simulink library "bynary_asteroid"  (R2015a)
settings: Solver=ode45  StartTime=0.0  StopTime=10.0  RelTol=1e-3
undefined symbols (not defined in the file or in its folder): Target
libraries: vrlib x3, lib_gravity x2, RotationalDynamics x2, TranslationalDynamics3DoF x1
settings Model: Creator=bbrito  LastModifiedBy=bbrito

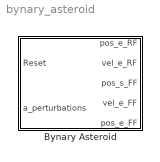
== system bynary_asteroid ==
  Bynary Asteroid : Subsystem  TreatAsAtomicUnit=on  mask{sphere=0, rt=0, ellip=0, sc=0, g=0, w0=0}
      mask prompts: sphere "Sphere parameters"; rt "Distance between bodies"; ellip "Ellipsoid parameters"; sc "Spacecraft initial conditions"; g "Gravitational constant"; w0 "Rotational speed"

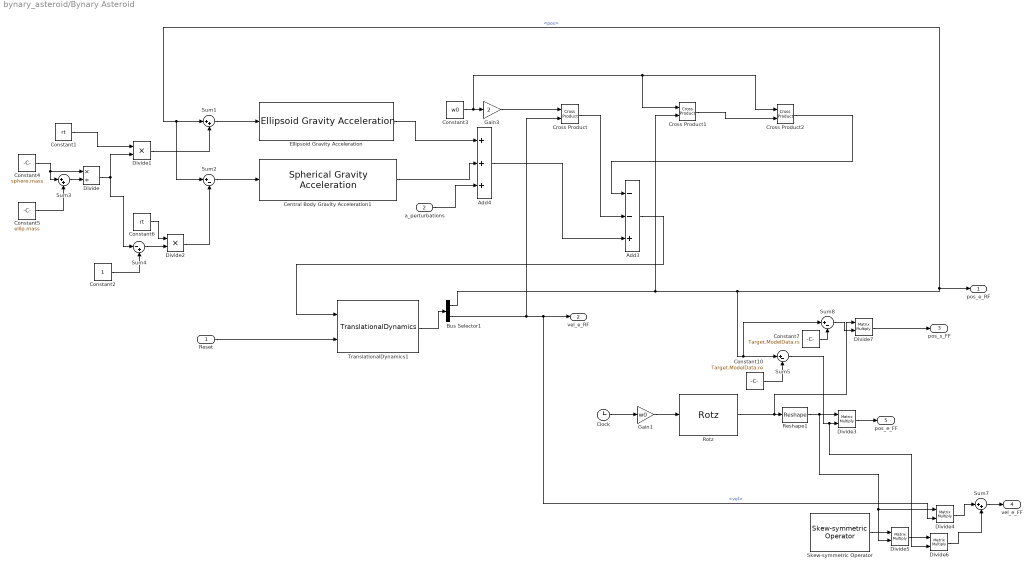
== system bynary_asteroid/Bynary Asteroid ==
  Reset : Inport
  a_perturbations : Inport  Port=2
  Add3 : Sum  Inputs=--+
  Add4 : Sum  Inputs=+++
  Bus Selector1 : BusSelector  OutputSignals=pos,vel
  Central Body Gravity Acceleration1 : lib_gravity/Spherical Gravity Acceleration  u=sphere.mass*g
  Clock : Clock
  Constant1 : Constant  Value=rt
  Constant10 : Constant  Value=Target.ModelData.re
  Constant2 : Constant
  Constant3 : Constant  Value=w0
  Constant4 : Constant  Value=sphere.mass
  Constant5 : Constant  Value=ellip.mass
  Constant6 : Constant  Value=rt
  Constant7 : Constant  Value=Target.ModelData.rs
  Cross Product : vrlib/Utilities/Cross Product
  Cross Product1 : vrlib/Utilities/Cross Product
  Cross Product2 : vrlib/Utilities/Cross Product
  Divide : Product  Inputs=*/
  Divide1 : Product  Inputs=**
  Divide2 : Product  Inputs=**
  Divide{3..7} (5 alike) : Product  Inputs=**  Multiplication=Matrix(*)
  Ellipsoid Gravity Acceleration : lib_gravity/Ellipsoid Gravity Acceleration  dim=ellip.dim  r0=ellip.r0  u=ellip.mass*g
  Gain1 : Gain  Gain=w0
  Gain3 : Gain  Gain=2
  Reshape1 : Reshape  OutputDimensionality=Customize  OutputDimensions=[3,3]
  Rotz : RotationalDynamics/Rotz
  Skew-symmetric Operator : RotationalDynamics/Skew-symmetric Operator  omega=Target.ModelData.Secondary.Rotation.w0
  Sum1 : Sum  Inputs=|++
  Sum2 : Sum  Inputs=|+-
  Sum3 : Sum  Inputs=|++
  Sum4 : Sum  Inputs=|-+
  Sum5 : Sum  Inputs=|+-
  Sum7 : Sum  Inputs=|++
  Sum8 : Sum  Inputs=|+-
  TranslationalDynamics1 : TranslationalDynamics3DoF/TranslationalDynamics  v0=sc.v0  x0=sc.x0
  pos_e_RF : Outport
  vel_e_RF : Outport  Port=2
  pos_s_FF : Outport  Port=3
  vel_e_FF : Outport  Port=4
  pos_e_FF : Outport  Port=5
  wires:
  Gain3/1 -> Cross Product/1
  Constant3/1 -> Cross Product1/1, Cross Product2/1, Gain3/1
  Cross Product1/1 -> Cross Product2/2
  Cross Product2/1 -> Add3/1
  Cross Product/1 -> Add3/2
  Sum1/1 -> Ellipsoid Gravity Acceleration/1
  Central Body Gravity Acceleration1/1 -> Add4/2
  Add4/1 -> Add3/3
  Sum2/1 -> Central Body Gravity Acceleration1/1
  Ellipsoid Gravity Acceleration/1 -> Add4/1
  TranslationalDynamics1/1 -> Bus Selector1/1
  Bus Selector1/2 -> Divide4/2, vel_e_RF/1, Cross Product/2  "<vel>"
  Bus Selector1/1 -> Cross Product1/2, Sum8/1, Sum5/1, pos_e_RF/1, Sum2/1, Sum1/1  "<pos>"
  Add3/1 -> TranslationalDynamics1/1
  Constant4/1 -> Divide/1, Sum3/1
  Constant5/1 -> Sum3/2
  Sum3/1 -> Divide/2
  Divide1/1 -> Sum1/2
  Divide/1 -> Sum4/1, Divide1/2
  Constant1/1 -> Divide1/1
  Constant2/1 -> Sum4/2
  Sum4/1 -> Divide2/2
  Constant6/1 -> Divide2/1
  Divide2/1 -> Sum2/2
  Reset/1 -> TranslationalDynamics1/2
  Rotz/1 -> Divide7/1, Reshape1/1
  Reshape1/1 -> Divide4/1, Divide5/2, Divide3/1
  Sum5/1 -> Divide6/2, Divide3/2
  Constant10/1 -> Sum5/2
  Divide3/1 -> pos_e_FF/1
  Skew-symmetric Operator/1 -> Divide5/1
  Divide5/1 -> Divide6/1
  Divide4/1 -> Sum7/1
  Divide6/1 -> Sum7/2
  Sum7/1 -> vel_e_FF/1
  Constant7/1 -> Sum8/2
  Divide7/1 -> pos_s_FF/1
  Sum8/1 -> Divide7/2
  Clock/1 -> Gain1/1
  Gain1/1 -> Rotz/1
  a_perturbations/1 -> Add4/3
